simulink model "rtwdemo_slbus"  (Simulink 7.6)
settings: Solver=FixedStepDiscrete  StartTime=0.0  StopTime=1  FixedStep=0.001  RelTol=1e-3
PostLoadFcn:
  | rtwdemo_slbus_data
libraries: rtwdemowidgets x3
Description:
  | Structure Definitions for Simulink(R) Bus Signals
settings Model: Creator=The MathWorks Inc.  ExtModeAutoUpdateStatusClock=off
settings MATStruct: SampleTime=0.001  Offset=0  Priority=[20.0]
settings DataIOCC: SaveOutput=off  SaveTime=off
settings OptimizationCC: InlineParams=on  InlineInvariantSignals=on  StateBitsets=on  DataBitsets=on  UseTempVars=on  EfficientFloat2IntCast=on  EfficientMapNaN2IntZero=off
settings DebuggingCC: CheckExecutionContextPreStartOutputMsg=on  CheckExecutionContextRuntimeOutputMsg=on  StrictBusMsg=ErrorOnBusTreatedAsVector
settings HardwareCC: ProdIntDivRoundTo=Zero  ProdEndianess=LittleEndian  ProdHWDeviceType=Generic->32-bit Embedded Processor  TargetHWDeviceType=Generic->32-bit Embedded Processor
settings RTWCC: Description=RTW Embedded Coder (no auto configuration)  GenerateReport=on  RTWVerbose=off  ProcessScript=grt_make_rtw_hook  LaunchReport=on
settings CodeAppCC: ForceParamTrailComments=on
settings GRTTargetCC: TargetFcnLib=ansi_tfl_tmw.mat

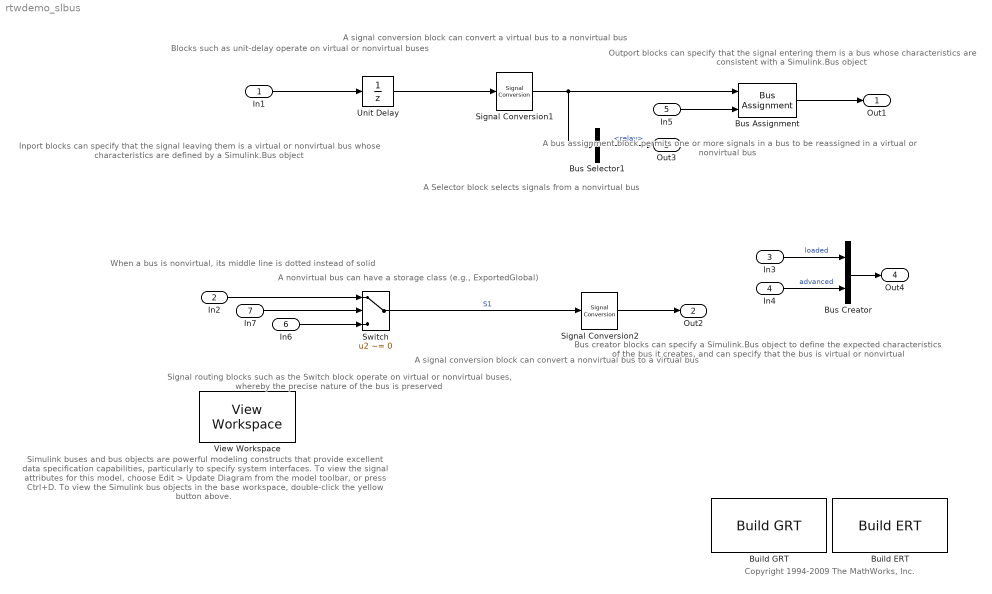
== system rtwdemo_slbus ==
  note: Blocks such as unit-delay operate
      | on virtual or nonvirtual buses
  note: A signal conversion block  can convert
      | a virtual bus to a nonvirtual bus
  note: A bus assignment block permits one or
      | more signals in a bus to be reassigned
      | in a virtual or nonvirtual bus
  note: Outport blocks can specify that
      | the signal entering them is a bus
      | whose characteristics are consistent
      | with a Simulink.Bus object
  note: Inport blocks can specify that
      | the signal leaving them is a
      | virtual or nonvirtual bus whose
      | characteristics are defined by a
      | Simulink.Bus object
  note: Signal routing blocks such
      | as the Switch block operate
      | on virtual or nonvirtual buses,
      | whereby the precise nature
      | of the bus is preserved
  note: A signal conversion block
      | can convert a nonvirtual
      | bus to a virtual bus
  note: A Selector block selects signals
      | from a nonvirtual bus
  note: When a bus is
      | nonvirtual, its middle line
      | is dotted instead of solid
  note: A nonvirtual bus can have a storage
      | class (e.g., ExportedGlobal)
  note: Simulink buses and bus objects are powerful modeling constructs that provide
      | excellent data specification capabilities, particularly to specify system interfaces.
      |
      | To view the signal attributes for this model, choose Edit > Update Diagram from
      | the model toolbar, or press Ctrl+D.  To view the Simulink bus objects in the base
      | workspace, double-click the yellow button above.
  note: Bus creator blocks can specify
      | a Simulink.Bus object to define the
      | expected characteristics of the bus it
      | creates, and can specify that the
      | bus is virtual or nonvirtual
  note: Copyright 1994-2009 The MathWorks, Inc.
  In1 : Inport  OutDataTypeStr=Bus: BusObject1
  In2 : Inport  Port=2  OutDataTypeStr=Bus: BusObject  BusOutputAsStruct=on
  In3 : Inport  Port=3  OutDataTypeStr=boolean  PortDimensions=1  SampleTime=0.001
  In4 : Inport  Port=4  OutDataTypeStr=boolean  PortDimensions=1  SampleTime=0.001
  In5 : Inport  Port=5  OutDataTypeStr=boolean  PortDimensions=1  SampleTime=0.001
  In6 : Inport  Port=6  OutDataTypeStr=Bus: BusObject  BusOutputAsStruct=on
  In7 : Inport  Port=7  OutDataTypeStr=boolean  PortDimensions=1  SampleTime=0.001
  Build ERT : rtwdemowidgets/Build ERT  SystemSampleTime=-1  attrib_overrides={}
  Build GRT : rtwdemowidgets/Build GRT  SystemSampleTime=-1  attrib_overrides={}
  Bus Creator : BusCreator  Inputs=2  OutDataTypeStr=Bus: BusObject2  NonVirtualBus=on
  Bus Selector1 : BusSelector  OutputSignals=relay
  Bus Assignment : BusAssignment  AssignedSignals=relay
  Signal Conversion1 : SignalConversion  ConversionOutput=Nonvirtual bus
  Signal Conversion2 : SignalConversion  ConversionOutput=Virtual bus
  Switch : Switch  Criteria=u2 ~= 0  ZeroCross=off
  Unit Delay : UnitDelay  SampleTime=0.001
  View Workspace : rtwdemowidgets/View Workspace  SystemSampleTime=-1
  Out1 : Outport  OutDataTypeStr=Bus: BusObject1
  Out2 : Outport  Port=2  OutDataTypeStr=Bus: BusObject
  Out3 : Outport  Port=3
  Out4 : Outport  Port=4  OutDataTypeStr=Bus: BusObject2
  wires:
  In1/1 -> Unit Delay/1
  Unit Delay/1 -> Signal Conversion1/1
  In2/1 -> Switch/1
  Switch/1 -> Signal Conversion2/1  "S1"
  Signal Conversion2/1 -> Out2/1
  Bus Selector1/1 -> Out3/1  "<relay>"
  Signal Conversion1/1 -> Bus Assignment/1, Bus Selector1/1
  Bus Assignment/1 -> Out1/1
  In5/1 -> Bus Assignment/2
  In6/1 -> Switch/3
  In7/1 -> Switch/2
  In3/1 -> Bus Creator/1  "loaded"
  In4/1 -> Bus Creator/2  "advanced"
  Bus Creator/1 -> Out4/1
